simulink model "taller6_bloques"  (R2020a)
settings: Solver=FixedStepAuto  StartTime=0.0  StopTime=35  FixedStep=0.001  RelTol=1e-3
settings Model: Creator=Personal  LastModifiedBy=Personal

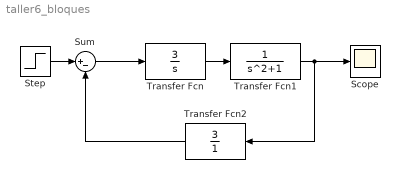
== system taller6_bloques ==
  Scope : Scope
  Step : Step  SampleTime=0
  Sum : Sum  Inputs=|+-
  Transfer Fcn : TransferFcn  Numerator=[3]  Denominator=[1 0]
  Transfer Fcn1 : TransferFcn  Denominator=[1 0 1]
  Transfer Fcn2 : TransferFcn  Numerator=[3]  Denominator=[0 1]
  wires:
  Transfer Fcn/1 -> Transfer Fcn1/1
  Sum/1 -> Transfer Fcn/1
  Transfer Fcn2/1 -> Sum/2
  Transfer Fcn1/1 -> Scope/1, Transfer Fcn2/1
  Step/1 -> Sum/1
